simulink model "sinus_model"  (Simulink 7.0)
settings: Solver=ode45  StartTime=0.0  StopTime=10.0  RelTol=1e-3
values from neighbouring files (symbols this model uses):
  a1 = -2*cos(f0*2*pi*Ts)    [cosinus.m]    (also in sinus.m)
  b0 = A    [cosinus.m]    (also in sinus.m = 0)
  b1 = -A*cos(f0*2*pi*Ts)    [cosinus.m]    (also in sinus.m = A*sin(f0*2*pi*Ts))
libraries: dspsigops x2
settings Model: Creator=fradet  LastModifiedBy=fradet

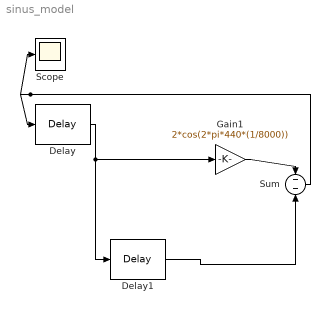
== system sinus_model ==
  Delay : dspsigops/Delay  dly_unit=Samples  delay=1  ic_detail=off  dif_ic_for_ch=off  dif_ic_for_dly=off  ic=0  reset_popup=None
  Delay1 : dspsigops/Delay  dly_unit=Samples  delay=1  ic_detail=off  dif_ic_for_ch=off  dif_ic_for_dly=off  ic=b1-b0*a1  reset_popup=None
  Gain1 : Gain  Gain=2*cos(2*pi*440*(1/8000))  ParameterDataType=sfix(16)  ParameterScaling=2^0  OutDataType=sfix(16)  OutScaling=2^0  SampleTime=1/8000
  Scope : Scope
  Sum : Sum  Inputs=--  OutDataType=sfix(16)  OutScaling=2^0  SampleTime=1/8000
  wires:
  Delay/1 -> Delay1/1, Gain1/1
  Delay1/1 -> Sum/2
  Sum/1 -> Scope/1, Delay/1
  Gain1/1 -> Sum/1
